simulink model "DAddConRA_AR"  (Simulink 7.8)
settings: Solver=ode45  StartTime=0.0  StopTime=10.0  RelTol=1e-3
settings Model: Creator=Arne Haber  LastModifiedBy=fkolass

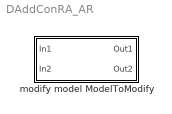
== system DAddConRA_AR ==
  modify model ModelToModify : Subsystem

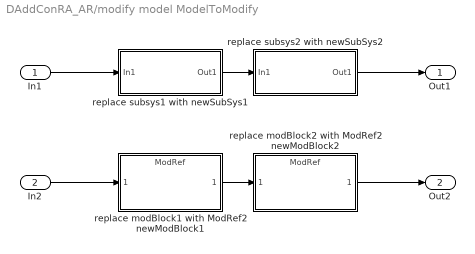
== system DAddConRA_AR/modify model ModelToModify ==
  In1 : Inport
  In2 : Inport  Port=2
  replace modBlock1 with ModRef2 newModBlock1 : ModelReference  ModelNameDialog=ModRef  SimulationMode=Normal  ModelReferenceVersion=1.2  CopyOfModelName=ModRef  DefaultDataLogging=on
  replace modBlock2 with ModRef2 newModBlock2 : ModelReference  ModelNameDialog=ModRef  SimulationMode=Normal  ModelReferenceVersion=1.2  CopyOfModelName=ModRef  DefaultDataLogging=on
  replace subsys1 with newSubSys1 : Subsystem
  replace subsys2 with newSubSys2 : Subsystem
  Out1 : Outport
  Out2 : Outport  Port=2
  wires:
  In1/1 -> replace subsys1 with newSubSys1/1(In1)
  replace subsys1 with newSubSys1/1(Out1) -> replace subsys2 with newSubSys2/1(In1)
  replace subsys2 with newSubSys2/1(Out1) -> Out1/1
  In2/1 -> replace modBlock1 with ModRef2 newModBlock1/1
  replace modBlock1 with ModRef2 newModBlock1/1 -> replace modBlock2 with ModRef2 newModBlock2/1
  replace modBlock2 with ModRef2 newModBlock2/1 -> Out2/1

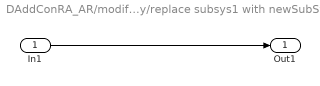
== system DAddConRA_AR/modify model ModelToModify/replace subsys1 with newSubSys1 ==
  In1 : Inport
  Out1 : Outport
  wires:
  In1/1 -> Out1/1

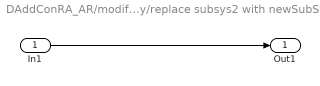
== system DAddConRA_AR/modify model ModelToModify/replace subsys2 with newSubSys2 ==
  In1 : Inport
  Out1 : Outport
  wires:
  In1/1 -> Out1/1
